simulink model "controller"  (R2026a)
settings: Solver=VariableStepAuto
undefined symbols (not defined in the file): Ctrl
libraries: aerolibutil x2, matrix_library x1, slpidlib x1
settings Model: Creator=arroy  LastModifiedBy=Owner

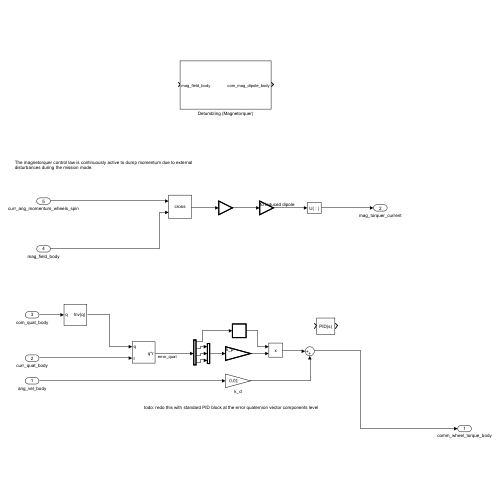
[thumbnail: Simulink's stored preview of the top-level diagram]
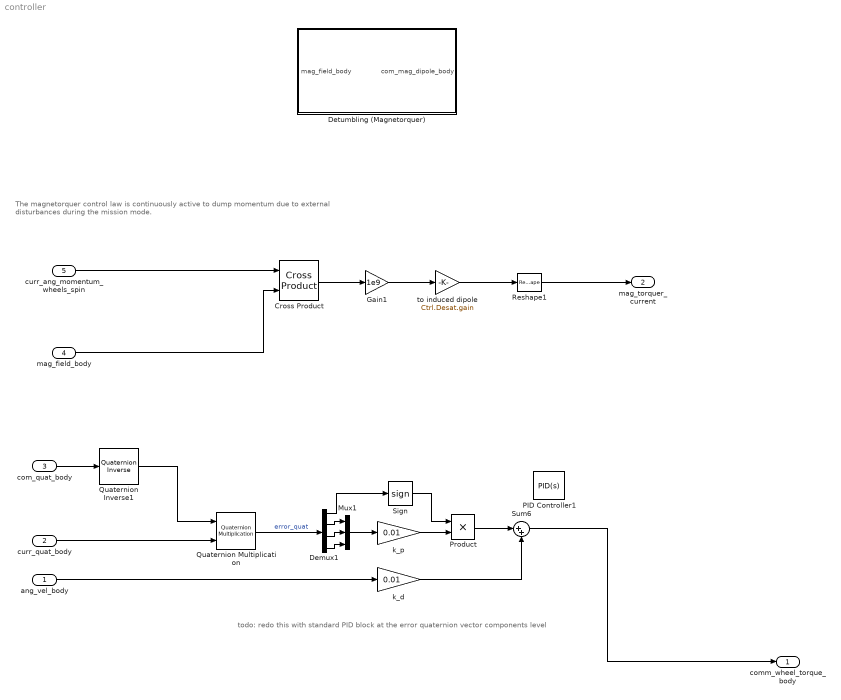
== system controller ==
  note: todo: redo this with standard PID block at the error quaternion vector components level
  note: The magnetorquer control law is continuously active to dump momentum due to external disturbances during the mission mode.
  ang_vel_body : Inport
  curr_quat_body : Inport  Port=2
  com_quat_body : Inport  Port=3
  mag_field_body : Inport  Port=4
  curr_ang_momentum_wheels_spin : Inport  Port=5
  Cross Product : matrix_library/Cross Product
  Demux1 : Demux
  Detumbling (Magnetorquer) : Subsystem
  Gain1 : Gain  Gain=1e9
  Mux1 : Mux  Inputs=3
  PID Controller1 : slpidlib/PID Controller  Controller=PID  Form=Parallel  TimeDomain=Continuous-time  UseExternalTs=off  SampleTime=-1  IntegratorMethod=Forward Euler  FilterMethod=Forward Euler  ControllerParametersSource=internal  P=Ctrl.PD.Kp  I=1  UseKiTs=on  D=Ctrl.PD.Kd  UseExternalDerivativeSource=off  N=100  UseFilter=on  TunerSelectOption=Transfer Function Based (PID Tuner App)  InitialConditionSource=internal  InitialConditionForIntegrator=0  InitialConditionForFilter=0  DifferentiatorICPrevScaledInput=0  ExternalReset=none  TrackingMode=off  Kt=1  LimitOutput=off  SatLimitsSource=internal  UpperSaturationLimit=inf  LowerSaturationLimit=-inf  LinearizeAsGain=on  AntiWindupMode=none  Kb=1  LimitIntegrator=off  UpperIntegratorSaturationLimit=inf  LowerIntegratorSaturationLimit=-inf  POutMin=[]  POutMax=[]  IOutMin=[]  IOutMax=[]  DOutMin=[]  DOutMax=[]  NOutMin=[]  NOutMax=[]  SumOutMin=[]  SumOutMax=[]  SaturationOutMin=[]  SaturationOutMax=[]  PParamMin=[]  PParamMax=[]  IParamMin=[]  IParamMax=[]  DParamMin=[]  DParamMax=[]  NParamMin=[]  NParamMax=[]  KbParamMin=[]  KbParamMax=[]  KtParamMin=[]  KtParamMax=[]  KbOutMin=[]  KbOutMax=[]  KtOutMin=[]  KtOutMax=[]  IntegratorOutMin=[]  IntegratorOutMax=[]  FilterOutMin=[]  FilterOutMax=[]  SumI1OutMin=[]  SumI1OutMax=[]  SumI2OutMin=[]  SumI2OutMax=[]  SumI3OutMin=[]  SumI3OutMax=[]  SumI4OutMin=[]  SumI4OutMax=[]  SumDOutMin=[]  SumDOutMax=[]  DifferentiatorOutMin=[]  DifferentiatorOutMax=[]  FilterDiffOutCoefMin=[]  FilterDiffOutCoefMax=[]  ReciprocalOutMin=[]  ReciprocalOutMax=[]  SumDenOutMin=[]  SumDenOutMax=[]  SumNumOutMin=[]  SumNumOutMax=[]  DivideOutMin=[]  DivideOutMax=[]  UdiffTsProdOutMin=[]  UdiffTsProdOutMax=[]  NTsProdOutMin=[]  NTsProdOutMax=[]  UintegralTsProdOutMin=[]  UintegralTsProdOutMax=[]  UngainTsProdOutMin=[]  UngainTsProdOutMax=[]  ClampingZeroOutDataTypeStr=Inherit: Inherit via back propagation  ClampingZeroOutMin=[]  ClampingZeroOutMax=[]  FilterDenConstantOutDataTypeStr=Inherit: Inherit via back propagation  FilterDenConstantOutMin=[]  FilterDenConstantOutMax=[]  PCopyOutDataTypeStr=Inherit: Inherit via back propagation  PCopyOutMin=[]  PCopyOutMax=[]  NCopyOutDataTypeStr=Inherit: Inherit via back propagation  NCopyOutMin=[]  NCopyOutMax=[]  IntegratorContinuousStateAttributes=''  IntegratorStateMustResolveToSignalObject=off  IntegratorRTWStateStorageClass=Auto  FilterContinuousStateAttributes=''  FilterStateMustResolveToSignalObject=off  FilterRTWStateStorageClass=Auto  ParallelPVariant=InternalParameters  IdealPVariant=Disabled  IVariant=InternalParameters  DVariant=InternalParameters  IntegratorVariant=Continuous  SatVariant=Disabled  AWVariant=Passthrough  PCopyVariant=Disabled  TRVariant=Disabled  FdbkBlocksVariant=Forward  IdealPFdbkVariant=Disabled  SatFdbkVariant=Disabled  DerivativeFilterVariant=ContFilter  NVariant=InternalParameters  NCopyVariant=Disabled  FilterICVariant=InternalICsFilter  IntegratorICVariant=InternalICs  ExternalResetVariant=Disabled  TRSumVariant=Passthrough  SumFdbkVariant=Disabled  SumVariant=Sum_PID  TsampFilterVariant=InternalTs  TsampNgainVariant=Passthrough  TsampIntegralVariant=Disabled_SignalSpec  ExternalSaturationOutDataTypeStr=Inherit: Same as second input  DerivativeSourceVariant=ErrorSignal  PreIntVariant=InternalPreInt
  Product : Product
  Quaternion Inverse1 : aerolibutil/Quaternion Inverse
  Quaternion Multiplication : aerolibutil/Quaternion Multiplication
  Reshape1 : Reshape
  Sign : Signum
  Sum6 : Sum  Inputs=|++
  k_d : Gain  Gain=0.01
  k_p : Gain  Gain=0.01
  to induced dipole : Gain  Gain=Ctrl.Desat.gain
  comm_wheel_torque_body : Outport
  mag_torquer_current : Outport  Port=2
  wires:
  k_d/1 -> Sum6/2
  k_p/1 -> Product/2
  Gain1/1 -> to induced dipole/1
  to induced dipole/1 -> Reshape1/1
  Demux1/2 -> Mux1/1
  curr_quat_body/1 -> Quaternion Multiplication/2
  com_quat_body/1 -> Quaternion Inverse1/1
  Reshape1/1 -> mag_torquer_current/1
  Cross Product/1 -> Gain1/1
  Demux1/4 -> Mux1/3
  Sign/1 -> Product/1
  mag_field_body/1 -> Cross Product/2
  Quaternion Inverse1/1 -> Quaternion Multiplication/1
  Demux1/1 -> Sign/1
  Mux1/1 -> k_p/1
  Sum6/1 -> comm_wheel_torque_body/1
  ang_vel_body/1 -> k_d/1
  Product/1 -> Sum6/1
  Demux1/3 -> Mux1/2
  Quaternion Multiplication/1 -> Demux1/1  "error_quat"
  curr_ang_momentum_wheels_spin/1 -> Cross Product/1

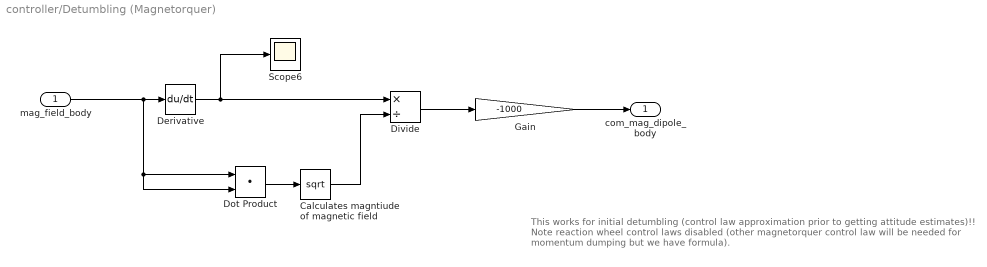
== system controller/Detumbling (Magnetorquer) ==
  note: This works for initial detumbling (control law approximation prior to getting attitude estimates)!! Note reaction wheel control laws disabled (other magnetorquer control law will be needed for momentum dumping but we have formula).
  mag_field_body : Inport
  Calculates magntiude of magnetic field : Sqrt
  Derivative : Derivative
  Divide : Product  Inputs=*/
  Dot Product : DotProduct  OutDataTypeStr=Inherit: Inherit via internal rule
  Gain : Gain  Gain=-1000
  Scope6 : Scope
      settings: ActiveDisplayYMinimum=-3E-7  ActiveDisplayYMaximum=3.2E-7  DataLoggingVariableName=ScopeData5
  com_mag_dipole_body : Outport
  wires:
  Derivative/1 -> Scope6/1, Divide/1
  mag_field_body/1 -> Dot Product/1, Dot Product/2, Derivative/1
  Divide/1 -> Gain/1
  Dot Product/1 -> Calculates magntiude of magnetic field/1
  Gain/1 -> com_mag_dipole_body/1
  Calculates magntiude of magnetic field/1 -> Divide/2
